simulink model "sampleModel1544"  (R2023a)
settings: Solver=VariableStepAuto  StartTime=0.0  StopTime=10.0  RelTol=1e-3
libraries: hdlsllib x4, simulink x2
settings Model: Creator=user1  LastModifiedBy=user1

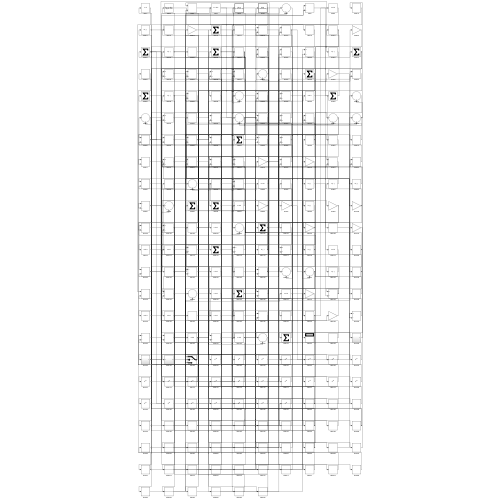
[thumbnail: Simulink's stored preview of the top-level diagram]
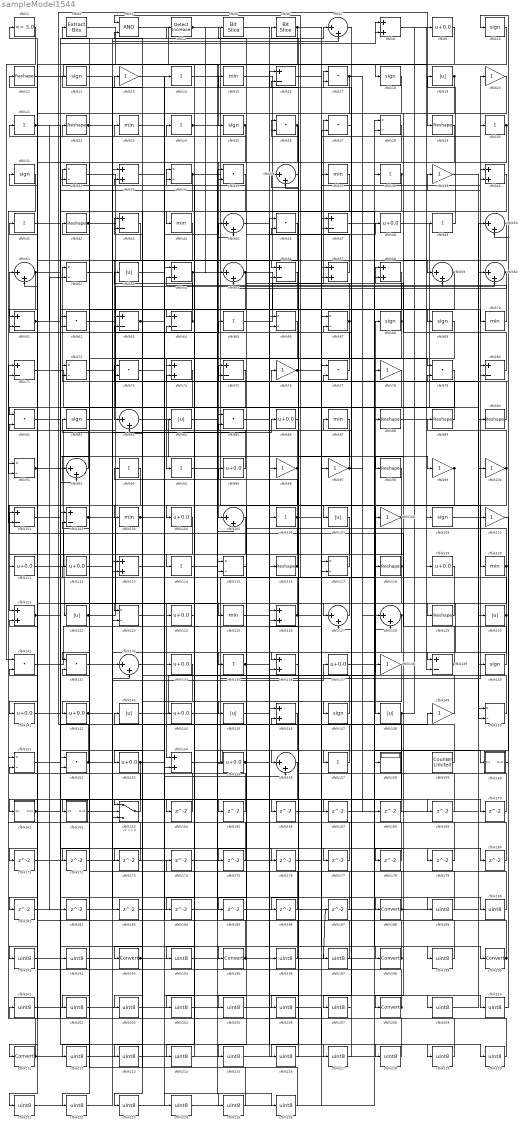
== system sampleModel1544 ==
  cfblk1 : hdlsllib/Logic and Bit Operations/Compare To Constant  relop=<=  const=3.0  OutDataTypeStr=boolean
  cfblk{10,12,18,25,31,68..69,82,109,140,147} (11 alike) : Signum
  cfblk{13,20,39,76,78,96..97,99..100,108,110,138,149} (13 alike) : Gain
  cfblk{16,43,47,56,61,63..64,71,75,80,101..102,139} (13 alike) : Sum  Inputs=+-
  cfblk{15,23,37,44,70,87,103,120,125} (9 alike) : MinMax
  cfblk{9,48,86,95,104,111..112,119,124,134,137,141..142,144,153,155} (16 alike) : Bias  Bias=0.0  SaturateOnIntegerOverflow=off
  cfblk{7,36,45,50..51,55,59..60,83,92,105,127..128,133,156} (15 alike) : Sum  Inputs=|++
  cfblk{14,21,24,30,38,41,49,65,93..94,106,114,135,157} (14 alike) : Sum  Inputs=+
  cfblk{19,53,84,107,122,130,143,145,148} (9 alike) : Abs  SaturateOnIntegerOverflow=off
  cfblk{11,22,29,42,88..90,98,116,118,129} (11 alike) : Reshape
  cfblk{8,33,40,54,57..58,74,113,121,126,136,146,154} (13 alike) : Sum
  cfblk{28,32,34,52,66..67,72,91,115,117,123,150..151} (13 alike) : Product  Inputs=*/  RndMeth=Zero  SaturateOnIntegerOverflow=on
  cfblk{17,26..27,35,46,62,73,77,79,81,85,131..132,152} (14 alike) : DotProduct  OutDataTypeStr=Inherit: Inherit via internal rule
  cfblk158 : Display
  cfblk159 : hdlsllib/Sources/Counter Limited  uplimit=7  tsamp=-1
  cfblk160 : Subsystem
      settings: LibrarySourceBlock=|
      | hdlsllib/Ports &
      | Subsystems/Subsystem
  cfblk161 : Subsystem
      settings: LibrarySourceBlock=|
      | hdlsllib/Ports &
      | Subsystems/Subsystem
  cfblk162 : Subsystem
      settings: LibrarySourceBlock=|
      | hdlsllib/Ports &
      | Subsystems/Subsystem
  cfblk163 : Switch  SaturateOnIntegerOverflow=off  InputSameDT=off
  cfblk{164..187} (24 alike) : Delay  SampleTime=1
  cfblk{188,193,195,198,200,208,211} (7 alike) : DataTypeConversion  SaturateOnIntegerOverflow=off  RndMeth=Floor
  cfblk{189..192,194,196..197,199,201..207,209..210,212..226} (32 alike) : DataTypeConversion  OutDataTypeStr=uint8  SaturateOnIntegerOverflow=off  RndMeth=Floor
  cfblk2 : simulink/Logic and Bit Operations/Extract Bits  bitsToExtract=Upper half  numBits=8  bitIdxRange=[0 7]  outScalingMode=Preserve fixed-point scaling
      settings: LibrarySourceBlock=|
      | hdlsllib/Logic and Bit
      | Operations/Extract Bits
  cfblk3 : Logic  AllPortsSameDT=off  OutDataTypeStr=boolean
  cfblk4 : simulink/Logic and Bit Operations/Detect Increase  vinit=0.0  OutDataTypeStr=boolean
      settings: LibrarySourceBlock=|
      | hdlsllib/Logic and Bit
      | Operations/Detect
      | Increase
  cfblk5 : hdlsllib/Logic and Bit Operations/Bit Slice  lidx=7  ridx=0
  cfblk6 : hdlsllib/Logic and Bit Operations/Bit Slice  lidx=7  ridx=0
  wires:
  cfblk136/1 -> cfblk44/1
  cfblk25/1 -> cfblk105/1, cfblk32/2, cfblk81/1, cfblk62/2
  cfblk119/1 -> cfblk129/1
  cfblk4/1 -> cfblk56/1, cfblk55/1
  cfblk143/1 -> cfblk68/1
  cfblk127/1 -> cfblk3/1
  cfblk118/1 -> cfblk82/1, cfblk181/1
  cfblk154/1 -> cfblk20/1
  cfblk148/1 -> cfblk9/1, cfblk212/1
  cfblk108/1 -> cfblk107/1, cfblk185/1
  cfblk122/1 -> cfblk80/1, cfblk86/1
  cfblk84/1 -> cfblk105/2
  cfblk24/1 -> cfblk117/1, cfblk197/1
  cfblk152/1 -> cfblk29/1, cfblk137/1, cfblk8/1
  cfblk28/1 -> cfblk211/1
  cfblk120/1 -> cfblk93/1, cfblk139/1
  cfblk116/1 -> cfblk21/1, cfblk73/1
  cfblk117/1 -> cfblk75/1
  cfblk1/1 -> cfblk131/1
  cfblk77/1 -> cfblk51/1
  cfblk69/1 -> cfblk94/1
  cfblk54/1 -> cfblk75/2, cfblk163/1
  cfblk110/1 -> cfblk155/1
  cfblk111/1 -> cfblk65/1
  cfblk65/1 -> cfblk27/1
  cfblk39/1 -> cfblk90/1
  cfblk15/1 -> cfblk97/1
  cfblk100/1 -> cfblk89/1, cfblk101/2
  cfblk37/1 -> cfblk153/1
  cfblk43/1 -> cfblk83/1
  cfblk99/1 -> cfblk148/1, cfblk186/1
  cfblk61/1 -> cfblk52/2, cfblk125/1, cfblk189/1
  cfblk32/1 -> cfblk140/1
  cfblk134/1 -> cfblk154/1
  cfblk36/1 -> cfblk6/1
  cfblk125/1 -> cfblk46/1
  cfblk135/1 -> cfblk210/1, cfblk215/1
  cfblk41/1 -> cfblk198/1
  cfblk7/1 -> cfblk157/1
  cfblk128/1 -> cfblk175/1, cfblk204/1
  cfblk129/1 -> cfblk127/1
  cfblk51/1 -> cfblk71/2, cfblk165/1
  cfblk11/1 -> cfblk18/1
  cfblk105/1 -> cfblk161/1(In1)
  cfblk33/1 -> cfblk195/1
  cfblk63/1 -> cfblk14/1, cfblk40/2
  cfblk10/1 -> cfblk64/1
  cfblk19/1 -> cfblk147/1, cfblk178/1
  cfblk92/1 -> cfblk31/1
  cfblk3/1 -> cfblk109/1
  cfblk58/1 -> cfblk117/2
  cfblk48/1 -> cfblk130/1
  cfblk76/1 -> cfblk30/1, cfblk199/1
  cfblk12/1 -> cfblk70/1
  cfblk159/1 -> cfblk143/1
  cfblk86/1 -> cfblk16/2
  cfblk88/1 -> cfblk119/1
  cfblk47/1 -> cfblk200/1
  cfblk104/1 -> cfblk141/1
  cfblk9/1 -> cfblk25/1
  cfblk62/1 -> cfblk100/1
  cfblk93/1 -> cfblk121/1
  cfblk138/1 -> cfblk193/1
  cfblk109/1 -> cfblk120/1
  cfblk91/1 -> cfblk122/1, cfblk99/1
  cfblk160/1(Out1) -> cfblk80/2
  cfblk35/1 -> cfblk104/1
  cfblk155/1 -> cfblk96/1, cfblk59/2, cfblk205/1
  cfblk82/1 -> cfblk76/1
  cfblk20/1 -> cfblk118/1
  cfblk53/1 -> cfblk45/1
  cfblk153/1 -> cfblk79/2, cfblk170/1, cfblk221/1
  cfblk89/1 -> cfblk52/1
  cfblk97/1 -> cfblk26/1, cfblk128/1
  cfblk141/1 -> cfblk102/1
  cfblk59/1 -> cfblk123/1, cfblk127/2
  cfblk26/1 -> cfblk74/1, cfblk216/1
  cfblk139/1 -> cfblk136/1, cfblk112/1
  cfblk74/1 -> cfblk123/2
  cfblk31/1 -> cfblk91/2
  cfblk38/1 -> cfblk114/1, cfblk103/1
  cfblk102/1 -> cfblk144/1, cfblk222/1
  cfblk42/1 -> cfblk126/2, cfblk172/1
  cfblk70/1 -> cfblk36/1
  cfblk95/1 -> cfblk12/1
  cfblk72/1 -> cfblk60/2
  cfblk163/1 -> cfblk102/2
  cfblk137/1 -> cfblk160/1(In1)
  cfblk8/1 -> cfblk49/1
  cfblk161/1(Out1) -> cfblk149/1, cfblk177/1
  cfblk29/1 -> cfblk98/1
  cfblk121/1 -> cfblk7/1, cfblk8/2
  cfblk68/1 -> cfblk22/1, cfblk134/1
  cfblk6/1 -> cfblk111/1, cfblk59/1
  cfblk17/1 -> cfblk61/1, cfblk57/2, cfblk168/1
  cfblk90/1 -> cfblk17/1
  cfblk2/1 -> cfblk115/2
  cfblk34/1 -> cfblk152/2, cfblk128/2
  cfblk55/1 -> cfblk162/1(In1), cfblk88/1, cfblk139/2, cfblk124/1, cfblk163/3, cfblk48/1
  cfblk57/1 -> cfblk24/1
  cfblk21/1 -> cfblk69/1, cfblk154/2, cfblk182/1
  cfblk145/1 -> cfblk106/1
  cfblk13/1 -> cfblk188/1
  cfblk144/1 -> cfblk38/1
  cfblk126/1 -> cfblk37/1, cfblk1/1
  cfblk49/1 -> cfblk19/1
  cfblk83/1 -> cfblk158/1
  cfblk22/1 -> cfblk7/2, cfblk56/2
  cfblk60/1 -> cfblk10/1, cfblk55/2
  cfblk142/1 -> cfblk17/2, cfblk4/1
  cfblk131/1 -> cfblk40/1
  cfblk81/1 -> cfblk39/1
  cfblk56/1 -> cfblk63/1
  cfblk14/1 -> cfblk45/2
  cfblk147/1 -> cfblk84/1
  cfblk52/1 -> cfblk79/1
  cfblk106/1 -> cfblk132/1, cfblk110/1, cfblk73/2
  cfblk98/1 -> cfblk145/1
  cfblk130/1 -> cfblk26/2, cfblk163/2
  cfblk115/1 -> cfblk95/1
  cfblk80/1 -> cfblk58/1
  cfblk30/1 -> cfblk156/1, cfblk202/1
  cfblk107/1 -> cfblk142/1
  cfblk157/1 -> cfblk43/1
  cfblk140/1 -> cfblk101/1
  cfblk16/1 -> cfblk108/1
  cfblk40/1 -> cfblk58/2
  cfblk149/1 -> cfblk85/2
  cfblk96/1 -> cfblk135/1, cfblk3/2
  cfblk50/1 -> cfblk208/1
  cfblk67/1 -> cfblk32/1, cfblk92/1, cfblk61/2, cfblk54/2
  cfblk71/1 -> cfblk150/2
  cfblk103/1 -> cfblk156/2, cfblk15/1
  cfblk150/1 -> cfblk72/1
  cfblk64/1 -> cfblk43/2, cfblk34/1
  cfblk75/1 -> cfblk164/1
  cfblk164/1 -> cfblk131/2
  cfblk165/1 -> cfblk2/1
  cfblk132/1 -> cfblk166/1
  cfblk166/1 -> cfblk150/1
  cfblk45/1 -> cfblk167/1
  cfblk167/1 -> cfblk67/2
  cfblk168/1 -> cfblk36/2
  cfblk123/1 -> cfblk169/1
  cfblk169/1 -> cfblk16/1
  cfblk170/1 -> cfblk126/1
  cfblk79/1 -> cfblk171/1
  cfblk171/1 -> cfblk115/1
  cfblk172/1 -> cfblk35/2
  cfblk156/1 -> cfblk173/1
  cfblk173/1 -> cfblk91/1
  cfblk174/1 -> cfblk77/1
  cfblk175/1 -> cfblk64/2
  cfblk162/1(Out1) -> cfblk176/1
  cfblk176/1 -> cfblk27/2
  cfblk177/1 -> cfblk121/2
  cfblk178/1 -> cfblk71/1
  cfblk94/1 -> cfblk179/1
  cfblk179/1 -> cfblk51/2
  cfblk5/1 -> cfblk180/1
  cfblk180/1 -> cfblk152/1
  cfblk181/1 -> cfblk92/2
  cfblk182/1 -> cfblk136/2
  cfblk112/1 -> cfblk183/1
  cfblk124/1 -> cfblk184/1
  cfblk184/1 -> cfblk60/1
  cfblk186/1 -> cfblk72/2
  cfblk187/1 -> cfblk34/2
  cfblk188/1 -> cfblk35/1, cfblk74/2
  cfblk189/1 -> cfblk13/1
  cfblk133/1 -> cfblk190/1
  cfblk190/1 -> cfblk53/1
  cfblk46/1 -> cfblk191/1
  cfblk191/1 -> cfblk133/1
  cfblk101/1 -> cfblk192/1
  cfblk192/1 -> cfblk133/2
  cfblk193/1 -> cfblk187/1, cfblk67/1
  cfblk18/1 -> cfblk194/1
  cfblk194/1 -> cfblk138/1
  cfblk195/1 -> cfblk83/2, cfblk54/1
  cfblk85/1 -> cfblk196/1
  cfblk196/1 -> cfblk33/1
  cfblk197/1 -> cfblk33/2
  cfblk198/1 -> cfblk81/2, cfblk85/1
  cfblk199/1 -> cfblk41/1
  cfblk200/1 -> cfblk46/2, cfblk5/1
  cfblk201/1 -> cfblk47/1
  cfblk202/1 -> cfblk47/2
  cfblk66/1 -> cfblk203/1
  cfblk203/1 -> cfblk63/2
  cfblk204/1 -> cfblk66/1
  cfblk205/1 -> cfblk66/2
  cfblk87/1 -> cfblk206/1
  cfblk27/1 -> cfblk207/1
  cfblk207/1 -> cfblk87/1
  cfblk208/1 -> cfblk132/2, cfblk11/1
  cfblk183/1 -> cfblk209/1
  cfblk209/1 -> cfblk50/1
  cfblk210/1 -> cfblk50/2
  cfblk211/1 -> cfblk201/1, cfblk116/1
  cfblk212/1 -> cfblk28/1
  cfblk44/1 -> cfblk213/1
  cfblk213/1 -> cfblk28/2
  cfblk146/1 -> cfblk214/1
  cfblk214/1 -> cfblk174/1
  cfblk215/1 -> cfblk146/1
  cfblk216/1 -> cfblk146/2
  cfblk151/1 -> cfblk217/1
  cfblk217/1 -> cfblk77/2
  cfblk206/1 -> cfblk218/1
  cfblk218/1 -> cfblk151/1
  cfblk185/1 -> cfblk219/1
  cfblk219/1 -> cfblk151/2
  cfblk113/1 -> cfblk220/1
  cfblk220/1 -> cfblk62/1
  cfblk221/1 -> cfblk113/1
  cfblk222/1 -> cfblk113/2
  cfblk78/1 -> cfblk223/1
  cfblk223/1 -> cfblk57/1
  cfblk73/1 -> cfblk224/1
  cfblk224/1 -> cfblk78/1
  cfblk23/1 -> cfblk225/1
  cfblk225/1 -> cfblk42/1
  cfblk114/1 -> cfblk226/1
  cfblk226/1 -> cfblk23/1

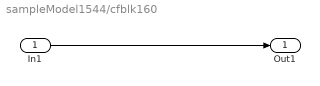
== system sampleModel1544/cfblk160 ==
  In1 : Inport
  Out1 : Outport
  wires:
  In1/1 -> Out1/1

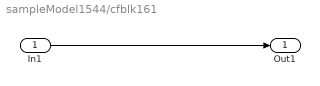
== system sampleModel1544/cfblk161 ==
  In1 : Inport
  Out1 : Outport
  wires:
  In1/1 -> Out1/1

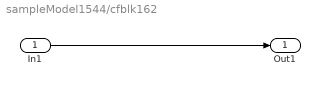
== system sampleModel1544/cfblk162 ==
  In1 : Inport
  Out1 : Outport
  wires:
  In1/1 -> Out1/1
